simulink model "mpsk_model2"  (Simulink 8.7)
settings: Solver=FixedStepDiscrete  StartTime=0.0  StopTime=2  FixedStep=ts  RelTol=1e-3  AbsTol=1e-6
PreLoadFcn:
  | fs=100000; ts=1/fs; R=1000; T=1/R; fc=10000; M=8;
libraries: commchan3 x2, commutil2 x1, simulink_extras x1, dspsrcs4 x1
settings Model: Creator=amoura  LastModifiedBy=Artur Moura
settings DataIOCC: LimitDataPoints=off  SignalLoggingSaveFormat=ModelDataLogs
settings OptimizationCC: BlockReduction=off  BooleanDataType=off  ExpressionDepthLimit=2147483647  InitFltsAndDblsToZero=on
settings DebuggingCC: SaveWithParameterizedLinksMsg=none  SignalResolutionControl=TryResolveAllWithWarning  MultiTaskDSMMsg=warning  MultiTaskCondExecSysMsg=none  FcnCallInpInsideContextMsg=UseLocalSettings  StateNameClashWarn=warning
settings HardwareCC: TargetUnknown=on
settings RTWCC: TemplateMakefile=grt_unix.tmf
settings GRTTargetCC: TargetFcnLib=ansi_tfl_tmw.mat  ModelReferenceCompliant=off  CombineOutputUpdateFcns=off  MatFileLogging=off  GRTInterface=on

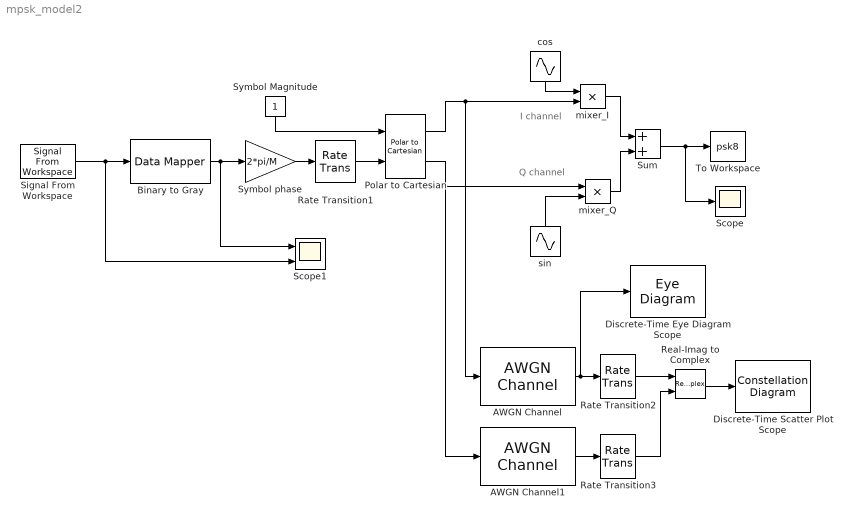
== system mpsk_model2 ==
  note: I channel
  note: Q channel
  AWGN Channel : commchan3/AWGN Channel  InputProcessing=Inherited (this choice will be removed - see release notes)  seed=67  noiseMode=Variance from mask  EbNodB=10  EsNodB=10  SNRdB=10  bitsPerSym=1  Ps=1  Tsym=1  variance=.001
  AWGN Channel1 : commchan3/AWGN Channel  InputProcessing=Inherited (this choice will be removed - see release notes)  seed=23  noiseMode=Variance from mask  EbNodB=10  EsNodB=10  SNRdB=10  bitsPerSym=1  Ps=1  Tsym=1  variance=.001
  Binary to Gray : commutil2/Data Mapper  MapMode=Binary to Gray  M=8  MapVec=[0 1 3 2 7 6 4 5]
  Discrete-Time Eye Diagram Scope : EyeDiagram  Tag=EyeDiagram
  Discrete-Time Scatter Plot Scope : ConstellationDiagram  Tag=ScatterPlot
  Polar to Cartesian : simulink_extras/Transformations/Polar to Cartesian
  Rate Transition1 : RateTransition  OutPortSampleTime=ts
  Rate Transition2 : RateTransition  OutPortSampleTime=1/1000
  Rate Transition3 : RateTransition  OutPortSampleTime=1/1000
  Real-Imag to Complex : RealImagToComplex  SampleTime=1/1000
  Scope : Scope
  Scope1 : Scope  NumInputPorts=2
  Signal From Workspace : dspsrcs4/Signal From Workspace  X=randi([0 7],10000,1)  Ts=1/1000  nsamps=1  OutputAfterFinalValue=Cyclic repetition  ignoreOrWarnInputAndFrameLengths=off  OutputFrames=on
  Sum : Sum  SampleTime=ts  SaturateOnIntegerOverflow=on  InputSameDT=on  OutDataTypeStr=Inherit: Same as first input
  Symbol Magnitude : Constant  SampleTime=ts
  Symbol phase : Gain  Gain=2*pi/M  SampleTime=1/1000  SaturateOnIntegerOverflow=on  OutDataTypeStr=Inherit: Same as input  ParamDataTypeStr=Inherit: Same as input
  To Workspace : ToWorkspace  VariableName=psk8  SampleTime=ts
  cos : Sin  Frequency=2*pi*fc  Phase=pi/2  SampleTime=0
  mixer_I : Product  SampleTime=ts  SaturateOnIntegerOverflow=on  RndMeth=Zero  InputSameDT=on  OutDataTypeStr=Inherit: Same as first input
  mixer_Q : Product  SampleTime=ts  SaturateOnIntegerOverflow=on  RndMeth=Zero  InputSameDT=on  OutDataTypeStr=Inherit: Same as first input
  sin : Sin  Frequency=2*pi*fc  SampleTime=0
  wires:
  Binary to Gray/1 -> Symbol phase/1, Scope1/1
  Signal From Workspace/1 -> Binary to Gray/1, Scope1/2
  Symbol Magnitude/1 -> Polar to Cartesian/1
  Symbol phase/1 -> Rate Transition1/1
  mixer_I/1 -> Sum/1
  mixer_Q/1 -> Sum/2
  sin/1 -> mixer_Q/2
  cos/1 -> mixer_I/1
  Sum/1 -> To Workspace/1, Scope/1
  Real-Imag to Complex/1 -> Discrete-Time Scatter Plot Scope/1
  Rate Transition1/1 -> Polar to Cartesian/2
  Polar to Cartesian/1 -> mixer_I/2, AWGN Channel/1
  Polar to Cartesian/2 -> AWGN Channel1/1, mixer_Q/1
  AWGN Channel/1 -> Rate Transition2/1, Discrete-Time Eye Diagram Scope/1
  AWGN Channel1/1 -> Rate Transition3/1
  Rate Transition2/1 -> Real-Imag to Complex/1
  Rate Transition3/1 -> Real-Imag to Complex/2
